simulink library "rotatingFoilCLCD"  (R2020a)
settings: Solver=VariableStepAuto  StartTime=0.0  StopTime=10.0  RelTol=1e-3
undefined symbols (not defined in the file or in its folder): aSurf
settings Model: Creator=jcreed2  LastModifiedBy=andre

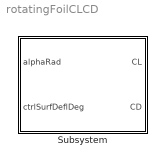
== system rotatingFoilCLCD ==
  Subsystem : Subsystem  mask{aSurf=aSurf}
      mask prompts: aSurf "Aerosurface Object"
      mask DialogControl DescGroupVar Prompt: Aerosurface CL/CD Calculator
      mask DialogControl DescTextVar Prompt: Define an aerosurface and included incidence angle. Subsystem computes CL/CD for the aerosurface under the apparent flow conditions.

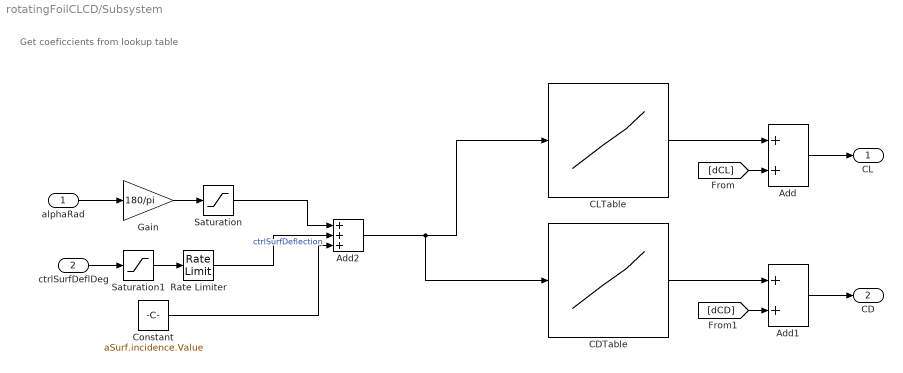
== system rotatingFoilCLCD/Subsystem ==
  note: Get coeficcients from lookup table
  alphaRad : Inport
  ctrlSurfDeflDeg : Inport  Port=2
  Add : Sum
  Add1 : Sum
  Add2 : Sum  Inputs=+++
  CDTable : Lookup_n-D  NumberOfTableDimensions=1  LookupTableObject=CLTable  BreakpointsForDimension1=aSurf.alpha.Value  Table=aSurf.CD.Value  ExtrapMethod=Clip  UseLastTableValue=on  InternalRulePriority=Speed  RndMeth=Simplest  InputSameDT=on
  CLTable : Lookup_n-D  NumberOfTableDimensions=1  LookupTableObject=CLTable  BreakpointsForDimension1=aSurf.alpha.Value  Table=aSurf.CL.Value  ExtrapMethod=Clip  UseLastTableValue=on  InternalRulePriority=Speed  RndMeth=Simplest  InputSameDT=on
  Constant : Constant  Value=aSurf.incidence.Value
  Gain : Gain  Gain=180/pi
  Rate Limiter : RateLimiter  RisingSlewLimit=aSurf.maxCtrlDefSpeed.Value  FallingSlewLimit=-aSurf.maxCtrlDefSpeed.Value  SampleTimeMode=inherited
  Saturation : Saturate  UpperLimit=90  LowerLimit=-90
  Saturation1 : Saturate  UpperLimit=aSurf.maxCtrlDef.Value  LowerLimit=aSurf.minCtrlDef.Value
  CL : Outport  VectorParamsAs1DForOutWhenUnconnected=off
  CD : Outport  Port=2  VectorParamsAs1DForOutWhenUnconnected=off
  wires:
  [dCL] -> Add/2
  CDTable/1 -> Add1/1
  Saturation/1 -> Add2/1
  alphaRad/1 -> Gain/1
  Add/1 -> CL/1
  Gain/1 -> Saturation/1
  Add1/1 -> CD/1
  CLTable/1 -> Add/1
  [dCD] -> Add1/2
  ctrlSurfDeflDeg/1 -> Saturation1/1
  Saturation1/1 -> Rate Limiter/1
  Add2/1 -> CDTable/1, CLTable/1
  Rate Limiter/1 -> Add2/2  "ctrlSurfDeflection"
  Constant/1 -> Add2/3
